simulink model "slrt_filelog_smoke"  (R2023b)
settings: Solver=FixedStepDiscrete  StartTime=0.0  StopTime=30  FixedStep=0.001  RelTol=1e-3
undefined symbols (not defined in the file or in its folder): DiscIntNeverNeededParam
libraries: slrealtimeloglib x4
settings Model: Creator=Administrator  LastModifiedBy=Administrator
settings SolverCC: ConcurrentTasks=on  PositivePriorityOrder=on
settings OptimizationCC: BlockReduction=off  OptimizeBlockIOStorage=off
settings DebuggingCC: TasksWithSamePriorityMsg=none
settings HardwareCC: ProdBitPerLong=64  ProdLongLongMode=on  ProdHWDeviceType=Intel->x86-64 (Linux 64)
settings RTWCC: Description=Simulink Real-Time  SystemTargetFile=slrealtime.tlc  TemplateMakefile=slrealtime_default_tmf  Toolchain=Simulink Real-Time Toolchain  BuildConfiguration=Faster Runs  CodeExecutionProfiling=on  TargetLang=C++
settings SimulinkRealTimeTargetCC: SLRTFileLogMaxRuns=5

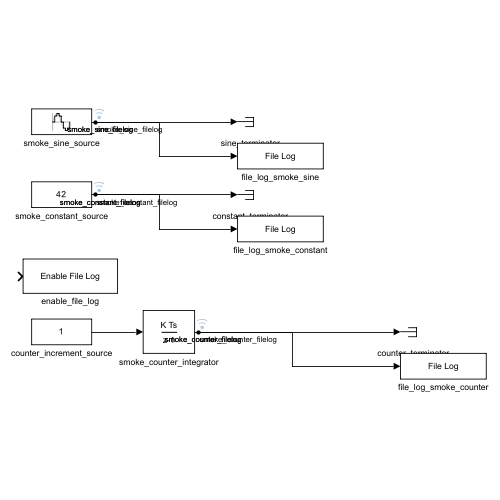
[thumbnail: Simulink's stored preview of the top-level diagram]
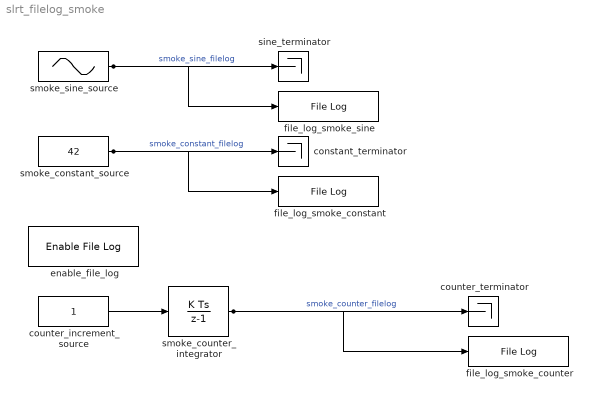
== system slrt_filelog_smoke ==
  constant_terminator : Terminator
  counter_increment_source : Constant
  counter_terminator : Terminator
  enable_file_log : slrealtimeloglib/Enable File Log
  file_log_smoke_constant : slrealtimeloglib/File Log  decimation=10  inputProcessing=Elements as channels (sample based)
  file_log_smoke_counter : slrealtimeloglib/File Log  decimation=10  inputProcessing=Elements as channels (sample based)
  file_log_smoke_sine : slrealtimeloglib/File Log  decimation=10  inputProcessing=Elements as channels (sample based)
  sine_terminator : Terminator
  smoke_constant_source : Constant  Value=42
  smoke_counter_integrator : DiscreteIntegrator  gainval=0.001  SampleTime=0.001  ICPrevOutput=DiscIntNeverNeededParam  ICPrevScaledInput=DiscIntNeverNeededParam
  smoke_sine_source : Sin  Frequency=2*pi*1  SampleTime=0.001
  wires:
  smoke_sine_source/1 -> sine_terminator/1, file_log_smoke_sine/1  "smoke_sine_filelog"
  smoke_constant_source/1 -> constant_terminator/1, file_log_smoke_constant/1  "smoke_constant_filelog"
  counter_increment_source/1 -> smoke_counter_integrator/1
  smoke_counter_integrator/1 -> counter_terminator/1, file_log_smoke_counter/1  "smoke_counter_filelog"
